simulink model "problem9"  (R2020a)
settings: Solver=VariableStepAuto  StartTime=0.0  StopTime=0.2  RelTol=1e-3
libraries: simulink x6, powerlib x5
settings Model: Creator=Admin  LastModifiedBy=Admin

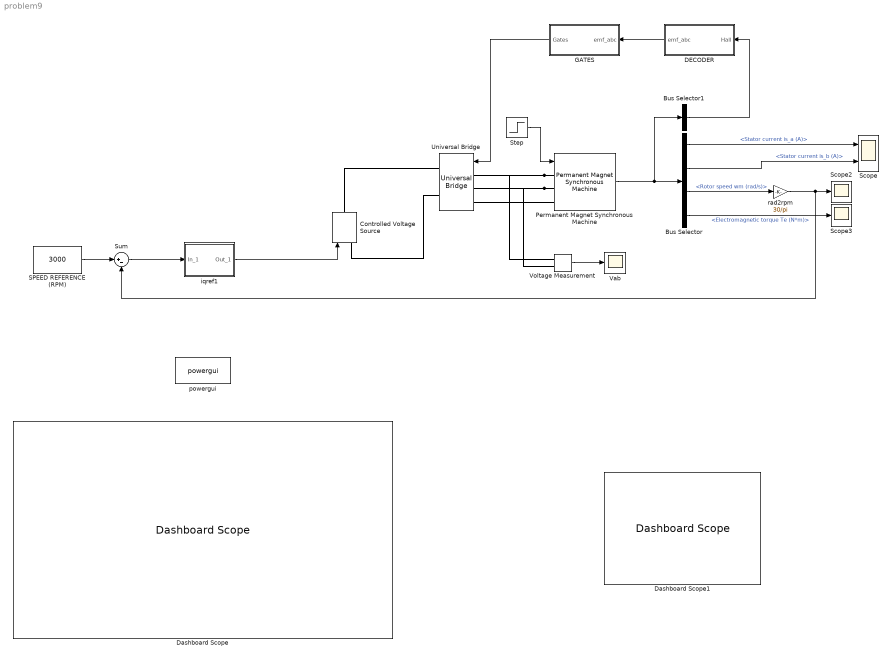
== system problem9 ==
  Bus Selector : BusSelector  OutputSignals=Stator current is_a (A),Stator current is_b (A),Rotor speed wm (rad/s),Electromagnetic torque Te (N*m)
  Bus Selector1 : BusSelector  OutputSignals=Hall effect signal h_a,Hall effect signal h_b,Hall effect signal h_c  OutputAsBus=on
  Controlled Voltage Source : powerlib/Electrical Sources/Controlled Voltage Source  Initialize=on  Source_Type=AC  Amplitude=0  Phase=0  Frequency=0  Measurements=None
  DECODER : Subsystem
  Dashboard Scope : DashboardScope
  Dashboard Scope1 : DashboardScope
  GATES : Subsystem
  Permanent Magnet Synchronous Machine : powerlib/Machines/Permanent Magnet Synchronous Machine  NbPhases=3  FluxDistribution=Trapezoidal  RotorType=Round  MechanicalLoad=Torque Tm  PresetModel=No  ShowDetailedParameters=on  MeasurementBus=off  Resistance=0.0485  Inductance=8.5e-3  dqInductances=[8.5e-3,8.5e-3]  La=0.000395  MachineConstant=Flux linkage established by magnets (V.s)  Flux=0.1194  VoltageCst=100.0283  TorqueCst=0.9552  Flat=120  Mechanical=[0.0027 0.0004924 4 0]  PolePairs=4  InitialConditions=[0,0, 0,0]  InitialConditions5ph=[0 0 0 0 0 0]  RefAngle=90 degrees behind phase A axis (modified Park)  IterativeDiscreteModel=Trapezoidal non iterative  TsBlock=-1  TsPowergui=0
  "SPEED REFERENCE (RPM) " : Constant  Value=3000
  Scope : Scope  NumInputPorts=2
  Scope2 : Scope
  Scope3 : Scope
  Step : Step  Time=0  SampleTime=0
  Sum : Sum  Inputs=|+-
  Universal Bridge : powerlib/Power Electronics/Universal Bridge  Arms=3  SnubberResistance=1e5  SnubberCapacitance=inf  Device=MOSFET / Diodes  Ron=1e-3  Lon=0  ForwardVoltages="[  0  0  ]"  ForwardVoltage=0  GTOparameters=[ 10e-6 , 20e-6 ]  IGBTparameters=[ 1e-6 , 2e-6 ]  Measurements=None  Measurements_2=None  converterType=Rectifier
  Vab : Scope
  Voltage Measurement : powerlib/Measurements/Voltage Measurement  PhasorSimulation=off  OutputType=Complex  PSBequivalent=0
  iqref1 : Subsystem  mask(PI Controller){I=16, P=0.013, sat=[-500, 500]}
      mask prompts: I "Integral"; P "Proportional:"; sat "Minimum and maximum outputs:"
      mask init:
      | min=sat(1);max=sat(2);
      mask Display: disp('PI')
  powergui : powerlib/powergui  Priority=1  SimulationMode=Discrete  SampleTime=50e-6  frequency=60  Iterations=50  frequencyindice=0  Pbase=100e6  ErrMax=1e-4  UnitsV=kV  UnitsW=MW  buscounter=0  FunctionMessages=off  echomessages=off  EnableUseOfTLC=off  CurrentSourceSwitches=off  DisableSnubberDevices=off  DisableRonSwitches=off  DisableVfSwitches=off  DisplayEquations=off  AutomaticDiscreteSolvers=off  SolverType=Tustin/Backward Euler (TBE)  Interpol=off  ExternalGateDelay=off  methode=off  Ts=100  x0status=blocks  SPID=on  SwTol=0  HookPort=off  NonlinearTolerance=0  nMaxIteration=15  ContinueOnMaxIteration=off  RestoreLinks=warning  ResistiveCurrentMeasurement=off  Frange=[0:2:500]  Ylog=off  Xlog=on  ShowGrid=off  save=off  variable=ZData  structure=0  ZoomFFT=off  StartTime=0.0  cycles=1  DisplayStyle=1  fundamental=60  FreqAxis=off  MaxFrequency=1000  frequencyindicesteady=1  RmsSteady=1  display=off
  rad2rpm : Gain  Gain=30/pi
  wires:
  Bus Selector1/1 -> DECODER/1("Hall ")
  Bus Selector/4 -> Scope3/1  "<Electromagnetic torque Te (N*m)>"
  Permanent Magnet Synchronous Machine/1 -> Bus Selector1/1, Bus Selector/1
  Sum/1 -> iqref1/1(In_1)
  iqref1/1(Out_1) -> Controlled Voltage Source/1
  "SPEED REFERENCE (RPM) "/1 -> Sum/1
  Bus Selector/3 -> rad2rpm/1  "<Rotor speed wm (rad/s)>"
  DECODER/1(emf_abc) -> GATES/1("emf_abc ")
  Step/1 -> Permanent Magnet Synchronous Machine/1
  GATES/1(Gates) -> Universal Bridge/1
  Voltage Measurement/1 -> Vab/1
  rad2rpm/1 -> Sum/2, Scope2/1
  Bus Selector/2 -> Scope/2  "<Stator current is_b (A)>"
  Bus Selector/1 -> Scope/1  "<Stator current is_a (A)>"
  connections:
  Permanent Magnet Synchronous Machine/LConn1 -- Universal Bridge/LConn1 -- Voltage Measurement/LConn1
  Permanent Magnet Synchronous Machine/LConn2 -- Universal Bridge/LConn2 -- Voltage Measurement/LConn2
  Universal Bridge/LConn3 -- Permanent Magnet Synchronous Machine/LConn3
  Controlled Voltage Source/RConn1 -- Universal Bridge/RConn1
  Controlled Voltage Source/LConn1 -- Universal Bridge/RConn2

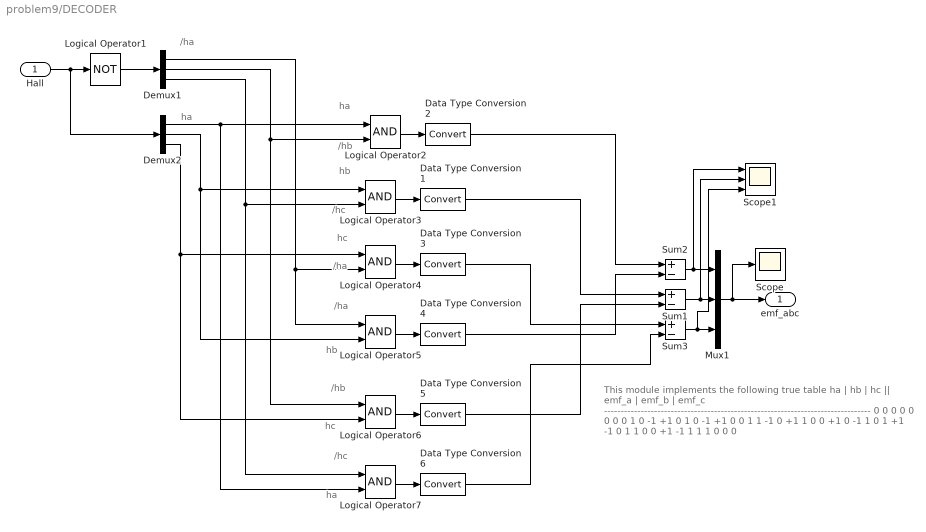
== system problem9/DECODER ==
  note: hc
  note: ha
  note: /ha
  note: hb
  note: hb
  note: /hb
  note: /hb
  note: /ha
  note: /hc
  note: ha
  note: This module implements the following true table
      |
      |    ha   |   hb   |   hc   ||   emf_a   |   emf_b   |   emf_c
      |     --------------------------------------------------------------------------------
      | 0          0         0          0               0               0
      | 0          0         1          0               -1              +1
      | 0          1         0          -1              +1                0
      | 0          1         1          -1               0               +1
      | 1          0         0         +1               0               -1
      | 1          0         1         +1              -1                0
      | 1          1         0          0              +1               -1
      | 1          1         1          0               0                0
  note: /ha
  note: /hc
  note: hc
  note: ha
  "Hall " : Inport
  Data Type Conversion{1..6} (6 alike) : DataTypeConversion
  Demux1 : Demux  Outputs=3
  Demux2 : Demux  Outputs=3
  Logical Operator1 : Logic  Operator=NOT  AllPortsSameDT=off  OutDataTypeStr=boolean
  Logical Operator{2..7} (6 alike) : Logic  AllPortsSameDT=off  OutDataTypeStr=boolean
  Mux1 : Mux  Inputs=3
  Scope : Scope
  Scope1 : Scope  NumInputPorts=3
  Sum1 : Sum  Inputs=+-  OutDataTypeStr=double
  Sum2 : Sum  Inputs=+-  OutDataTypeStr=double
  Sum3 : Sum  Inputs=+-  OutDataTypeStr=double
  emf_abc : Outport  VectorParamsAs1DForOutWhenUnconnected=off
  wires:
  Data Type Conversion2/1 -> Sum2/1
  Data Type Conversion3/1 -> Sum3/1
  Logical Operator5/1 -> Data Type Conversion4/1
  Mux1/1 -> Scope/1, emf_abc/1
  Logical Operator2/1 -> Data Type Conversion2/1
  Data Type Conversion1/1 -> Sum1/1
  Data Type Conversion4/1 -> Sum2/2
  Demux1/1 -> Logical Operator4/2, Logical Operator5/1
  Data Type Conversion6/1 -> Sum3/2
  Demux2/2 -> Logical Operator3/1, Logical Operator5/2
  Data Type Conversion5/1 -> Sum1/2
  Logical Operator1/1 -> Demux1/1
  "Hall "/1 -> Logical Operator1/1, Demux2/1
  Logical Operator4/1 -> Data Type Conversion3/1
  Logical Operator6/1 -> Data Type Conversion5/1
  Demux2/1 -> Logical Operator2/1, Logical Operator7/2
  Logical Operator3/1 -> Data Type Conversion1/1
  Demux2/3 -> Logical Operator4/1, Logical Operator6/2
  Logical Operator7/1 -> Data Type Conversion6/1
  Demux1/2 -> Logical Operator2/2, Logical Operator6/1
  Sum1/1 -> Scope1/2, Mux1/2
  Demux1/3 -> Logical Operator3/2, Logical Operator7/1
  Sum2/1 -> Scope1/1, Mux1/1
  Sum3/1 -> Scope1/3, Mux1/3

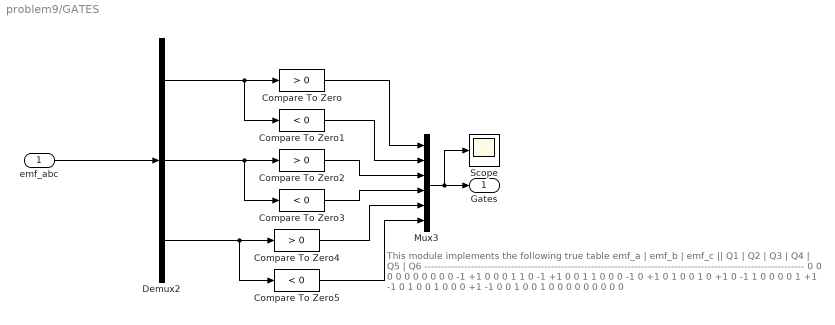
== system problem9/GATES ==
  note: This module implements the following true table
      |
      |    emf_a   |   emf_b   |   emf_c   ||   Q1   |   Q2   |   Q3   |   Q4   |   Q5   |   Q6
      |     ------------------------------------------------------------------------------------------------------------------
      |       0              0                0            0          0          0           0        0        0
      |       0               -1              +1          0          0          0           1        1        0
      |     -1              +1                0          0          1          1           0        0        0
      |     -1               0               +1          0          1         0           0        1        0
      |    +1               0                -1          1          0          0           0        0        1
      |    +1              -1                0           1          0          0           1        0        0
      |      0              +1               -1           0          0          1           0        0        1
      |     0              0                0             0          0          0           0        0        0
  "emf_abc " : Inport
  Compare To Zero : simulink/Logic and Bit Operations/Compare To Zero  relop=>  OutDataTypeStr=boolean  ZeroCross=off
  Compare To Zero1 : simulink/Logic and Bit Operations/Compare To Zero  relop=<  OutDataTypeStr=boolean  ZeroCross=off
  Compare To Zero2 : simulink/Logic and Bit Operations/Compare To Zero  relop=>  OutDataTypeStr=boolean  ZeroCross=off
  Compare To Zero3 : simulink/Logic and Bit Operations/Compare To Zero  relop=<  OutDataTypeStr=boolean  ZeroCross=off
  Compare To Zero4 : simulink/Logic and Bit Operations/Compare To Zero  relop=>  OutDataTypeStr=boolean  ZeroCross=off
  Compare To Zero5 : simulink/Logic and Bit Operations/Compare To Zero  relop=<  OutDataTypeStr=boolean  ZeroCross=off
  Demux2 : Demux  Outputs=3
  Mux3 : Mux  Inputs=6
  Scope : Scope
  Gates : Outport  VectorParamsAs1DForOutWhenUnconnected=off
  wires:
  Compare To Zero5/1 -> Mux3/6
  Demux2/2 -> Compare To Zero2/1, Compare To Zero3/1
  Compare To Zero3/1 -> Mux3/4
  Compare To Zero1/1 -> Mux3/2
  "emf_abc "/1 -> Demux2/1
  Demux2/3 -> Compare To Zero4/1, Compare To Zero5/1
  Compare To Zero/1 -> Mux3/1
  Compare To Zero2/1 -> Mux3/3
  Compare To Zero4/1 -> Mux3/5
  Mux3/1 -> Scope/1, Gates/1
  Demux2/1 -> Compare To Zero/1, Compare To Zero1/1

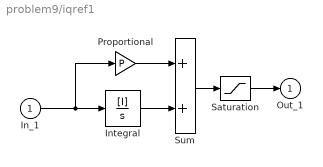
== system problem9/iqref1 ==
  In_1 : Inport
  Integral : TransferFcn  Numerator=[I]  Denominator=[1 0]
  Proportional : Gain  Gain=P  SaturateOnIntegerOverflow=on  OutDataTypeStr=Inherit: Same as input  ParamDataTypeStr=Inherit: Same as input
  Saturation : Saturate  UpperLimit=max  LowerLimit=min
  Sum : Sum  InputSameDT=on  SaturateOnIntegerOverflow=on  OutDataTypeStr=Inherit: Same as first input
  Out_1 : Outport  InitialOutput=0  VectorParamsAs1DForOutWhenUnconnected=off
  wires:
  Saturation/1 -> Out_1/1
  Sum/1 -> Saturation/1
  Proportional/1 -> Sum/1
  In_1/1 -> Proportional/1, Integral/1
  Integral/1 -> Sum/2
